simulink model "singleBiquadTestbench2_BAD"  (R2013b)
settings: Solver=ode45  StartTime=0.0  StopTime=120.0  RelTol=1e-3
undefined symbols (not defined in the file or in its folder): a, b, dfilt
libraries: dspvision x2, dsparch4 x1, dspsnks4 x1
settings Model: Creator=Preben  LastModifiedBy=Preben

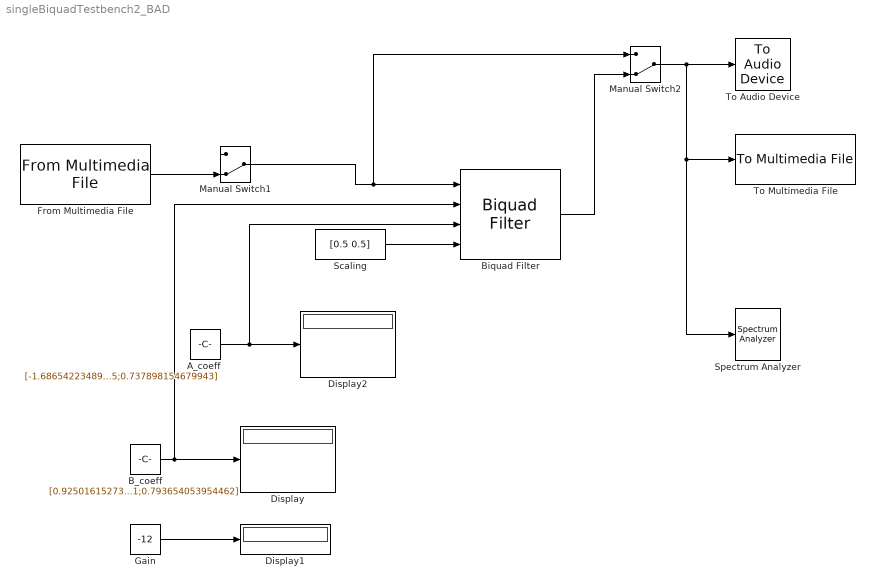
== system singleBiquadTestbench2_BAD ==
  A_coeff : Constant  Value=[-1.68654223489965;0.737898154679943]
  B_coeff : Constant  Value=[0.925016152739024;-1.7057701828861;0.793654053954462]
  Biquad Filter : dsparch4/Biquad Filter  IIRFiltStruct=Direct form II transposed  CoeffSource=Specify via dialog  BiQuadCoeffs=[b a]  a0Flag=Warning  IC=0  ICnum=0  ICden=0  denAccumFracLength=30  denProdOutputFracLength=30  secondMemoryFracLength=15  roundingMode=Floor  overflowMode=off  ScaleValues=1  optimizeScaleValues=on  ScaleValueMode=Specify via input port (g)  scaleValueFracLength=14  FilterSource=Input port(s)  dfiltObjectName=dfilt.df2tsos([1 0.3 0.4],[1 0.1 0.2])
  Display : Display
  Display1 : Display
  Display2 : Display
  From Multimedia File : dspvision/From Multimedia File  inputFilename=C:\Users\Preben\Dropbox\Matlab\Dat096\Audiofiles\07 Top Yourself_mono.wav  loop=on  numPlays=inf  outputStreams=Audio only  videoDataType=single  audioDataType=double  inheritSampleTime=on  userDefinedSampleTime=1/30  noAudioOutput=off  isIntensityVideo=off  fourcc=RGB  colorVideoFormat=Separate color signals  outputEOF=off  dataOrg=Column-major  audioFrameSize=1024  computeAudioFrameSize=off  outSamplingMode=Sample based
  Gain : Constant  Value=-12
  Manual Switch1 : ManualSwitch  CurrentSetting=0
  Manual Switch2 : ManualSwitch  CurrentSetting=0
  "Scaling " : Constant  Value=[0.5 0.5]
  Spectrum Analyzer : SpectrumAnalyzer
      settings: CopyFcn=scopeextensions.ScopeBlock.onCoreBlockCopy(gcbh);  DeleteFcn=scopeextensions.ScopeBlock.callback(gcbh, 'onBlockDelete');  PreSaveFcn=scopeextensions.ScopeBlock.callback(gcbh, 'onModelSave');  NameChangeFcn=scopeextensions.ScopeBlock.callback(gcbh, 'onBlockRename');  DestroyFcn=scopeextensions.ScopeBlock.onBlockDestroy(gcbh)  CloseFcn=scopeextensions.ScopeBlock.callback(gcbh, 'onBlockClose');  PreDeleteFcn=scopeextensions.ScopeBlock.callback(gcbh, 'onBlockPreDelete');
  To Audio Device : dspsnks4/To Audio Device  deviceName=ASIO Fireface USB  inheritSampleRate=on  sampleRate=44100  deviceDatatype=Determine from input data type  autoBufferSize=on  bufferSize=4096  queueDuration=1.0  defaultOutputChannelMapping=on  outputChannelMapping=1:18
  To Multimedia File : dspvision/To Multimedia File  outputFilename=output.wav  streamSelection=Audio only  videoCompressor=None (uncompressed)  audioCompressor=None (uncompressed)  imagePorts=Separate color signals  fileType=WAV  audioDatatype=16-bit integer  fourcc=RGB
  wires:
  Manual Switch2/1 -> To Multimedia File/1, Spectrum Analyzer/1, To Audio Device/1
  Biquad Filter/1 -> Manual Switch2/2
  B_coeff/1 -> Biquad Filter/2, Display/1
  Gain/1 -> Display1/1
  A_coeff/1 -> Biquad Filter/3, Display2/1
  "Scaling "/1 -> Biquad Filter/4
  From Multimedia File/1 -> Manual Switch1/2
  Manual Switch1/1 -> Manual Switch2/1, Biquad Filter/1
